simulink model "part4"  (R2016a)
settings: Solver=VariableStepAuto  StartTime=0.0  StopTime=10.0  RelTol=1e-3
libraries: simulink x2
settings Model: Creator=Administrator  LastModifiedBy=Administrator

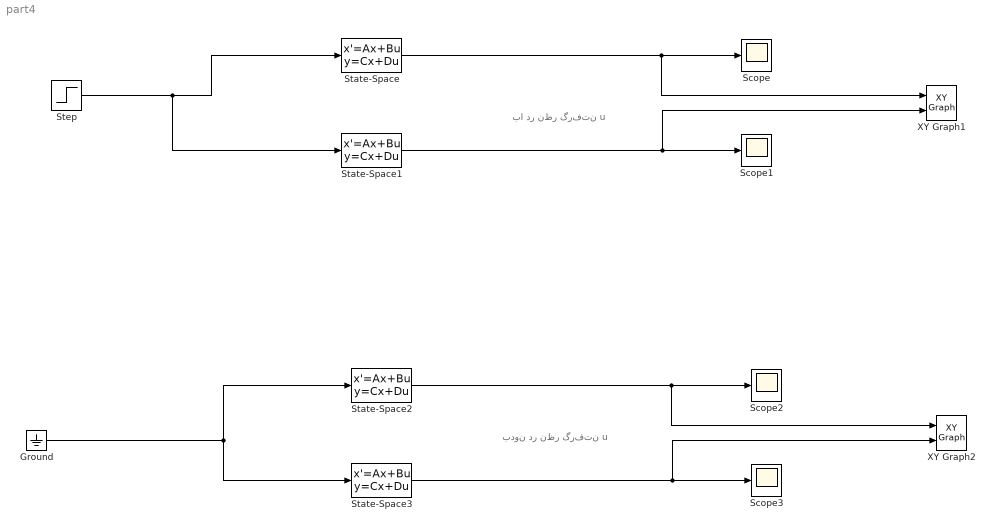
== system part4 ==
  note: بدون در نظر گرفتن u
  note: با در نظر گرفتن u
  Ground : Ground
  Scope{,1..3} (4 alike) : Scope
  State-Space : StateSpace  A=[0 -0.04; 0.3 0]  B=[1; 0]  C=[1 0]  D=0  X0=[0.1, 2]
  State-Space1 : StateSpace  A=[0 -0.04; 0.3 0]  B=[1; 0]  C=[0 1]  D=0  X0=[0.1, 2]
  State-Space2 : StateSpace  A=[0 -0.04; 0.3 0]  B=[0; 0]  C=[1 0]  D=0  X0=[0.1, 2]
  State-Space3 : StateSpace  A=[0 -0.04; 0.3 0]  B=[0; 0]  C=[0 1]  D=0  X0=[0.1, 2]
  Step : Step  SampleTime=0
  XY Graph1 : simulink/Sinks/XY Graph  xmin=-2  xmax=10  ymin=0  ymax=20  st=0.1
  XY Graph2 : simulink/Sinks/XY Graph  xmin=-2  xmax=10  ymin=0  ymax=3  st=0.1
  wires:
  State-Space/1 -> XY Graph1/1, Scope/1
  Step/1 -> State-Space1/1, State-Space/1
  State-Space1/1 -> XY Graph1/2, Scope1/1
  State-Space2/1 -> XY Graph2/1, Scope2/1
  State-Space3/1 -> XY Graph2/2, Scope3/1
  Ground/1 -> State-Space2/1, State-Space3/1
